simulink model "task1sim"  (R2022b)
settings: Solver=VariableStepAuto  StartTime=0.0  StopTime=6000  RelTol=1e-3
values from neighbouring files (symbols this model uses):
  A_1 = ( 1 / (C_1*C_2*R_2) )    (= 3.33333333333e-05)    [Task1.m]
  A_2 = (1/C_1)    (= 0.02)    [Task1.m]
  B_1 = 1    [Task1.m]
  B_2 = ( (1 / ( ((C_1)^2) * R_12 )) + (1 / (C_1*C_2*R_23)) )    (= 0.000146666666667)    [Task1.m]
  D_1 = ( (1 / (C_1*R_12)) + (1 / (C_2*R_23)))    (= 0.00733333333333)    [Task1.m]
  D_2 = (1 / ( ((C_1)^2)*C_2*R_12*R_23 ))    (= 2.66666666667e-07)    [Task1.m]
  E_1 = ( ( ((R_2)^2) - (R_12*R_23) ) / ( C_1*C_2*R_12*R_23*((R_2)^2) ) )    (= 1e-05)    [Task1.m]
  E_2 = 1    [Task1.m]
  F_2 = ( (2 / (C_1*R_12)) + (1 / (C_2*R_23)))    (= 0.0113333333333)    [Task1.m]
  G_2 = ( (1 / ( ((C_1)^2) * ((R_12)^2) )) + (1 / (C_1*C_2*R_12*R_23)) + ( (((R_2)^2) - (R_12*R_23)) / (C_1*C_2*R_12*R_23*((R_2)^2)) ) )    (= 3.93333333333e-05)    [Task1.m]
  H_2 = ( (((R_2)^2) - (R_12*R_23)) / ( ((C_1)^2)*C_2*((R_12)^2)*R_23*((R_2)^2)) )    (= 4e-08)    [Task1.m]
  theta_a = 293.15    [Task1.m]
settings Model: Creator=daddal  LastModifiedBy=daddal

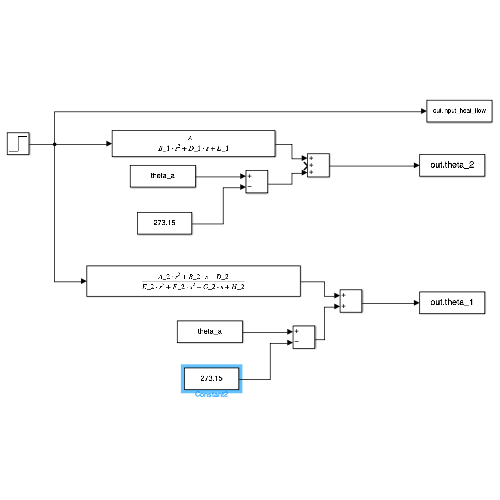
[thumbnail: Simulink's stored preview of the top-level diagram]
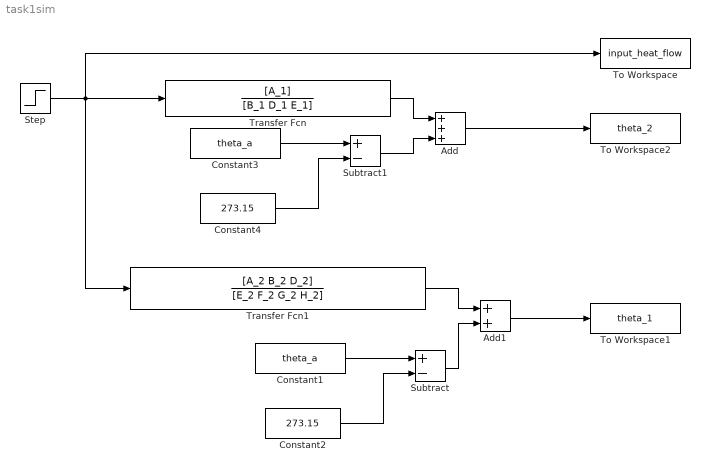
== system task1sim ==
  Add : Sum  Inputs=+++
  Add1 : Sum
  Constant1 : Constant  Value=theta_a
  Constant2 : Constant  Value=273.15
  Constant3 : Constant  Value=theta_a
  Constant4 : Constant  Value=273.15
  Step : Step  Time=600  After=3  SampleTime=0
  Subtract : Sum  Inputs=+-
  Subtract1 : Sum  Inputs=+-
  To Workspace : ToWorkspace  VariableName=input_heat_flow  SaveFormat=Timeseries  SampleTime=-1
  To Workspace1 : ToWorkspace  VariableName=theta_1  SaveFormat=Timeseries  SampleTime=-1
  To Workspace2 : ToWorkspace  VariableName=theta_2  SaveFormat=Timeseries  SampleTime=-1
  Transfer Fcn : TransferFcn  Numerator=[A_1]  Denominator=[B_1 D_1 E_1]
  Transfer Fcn1 : TransferFcn  Numerator=[A_2 B_2 D_2]  Denominator=[E_2 F_2 G_2 H_2]
  wires:
  Transfer Fcn/1 -> Add/1
  Step/1 -> To Workspace/1, Transfer Fcn1/1, Transfer Fcn/1
  Subtract1/1 -> Add/3
  Constant2/1 -> Subtract/2
  Subtract/1 -> Add1/2
  Transfer Fcn1/1 -> Add1/1
  Constant3/1 -> Subtract1/1
  Constant4/1 -> Subtract1/2
  Constant1/1 -> Subtract/1
  Add/1 -> To Workspace2/1
  Add1/1 -> To Workspace1/1
